simulink model "AC_FOC_PMSM_Developing_Rev_5"  (R2023b)
settings: Solver=VariableStepAuto  StartTime=0.0  StopTime=1  MaxStep=1e-4  RelTol=1e-3
values from neighbouring files (symbols this model uses):
  B = 11e-5    (= 0.00011)    [AB_FOC_For_PMSM_Parameters.m]
  Id_ref = 0    [AB_FOC_For_PMSM_Parameters.m]
  J = 0.47e-4    (= 4.7e-05)    [AB_FOC_For_PMSM_Parameters.m]
  Kcq = (2*zeta*wn*L) - Rs    (= 84.52)    [AB_FOC_For_PMSM_Parameters.m]
  Kcs = ((2*zeta*wns) - (B/J)) / ((1.5 *(pole^2)*flux)/J)    (= 0.00768666666667)    [AB_FOC_For_PMSM_Parameters.m]
  Ld = 7e-2    (= 0.07)    [AB_FOC_For_PMSM_Parameters.m]
  Lq = 7e-2    (= 0.07)    [AB_FOC_For_PMSM_Parameters.m]
  pole = 2    [AB_FOC_For_PMSM_Parameters.m]
  Rs = 2.98    [AB_FOC_For_PMSM_Parameters.m]
  speed_ref = 500    [AB_FOC_For_PMSM_Parameters.m]
libraries: fuzblock x10, slpidlib x9, spsDCVoltageSourceLib x5, spsPermanentMagnetSynchronousMachineLib x5, spsThreePhaseVIMeasurementLib x5, spsUniversalBridgeLib x5, spsdq0toabcLib x1, sps_lib x1
(part 1 of 2)
settings Model: Creator=hkurt  LastModifiedBy=hkurt
settings SolverCC: ZeroCrossAlgorithm=Adaptive

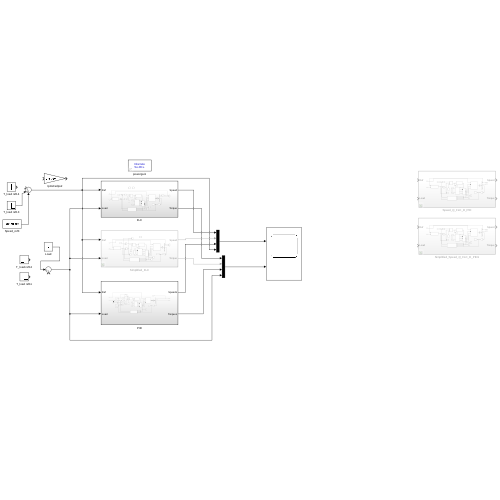
[thumbnail: Simulink's stored preview of the top-level diagram]
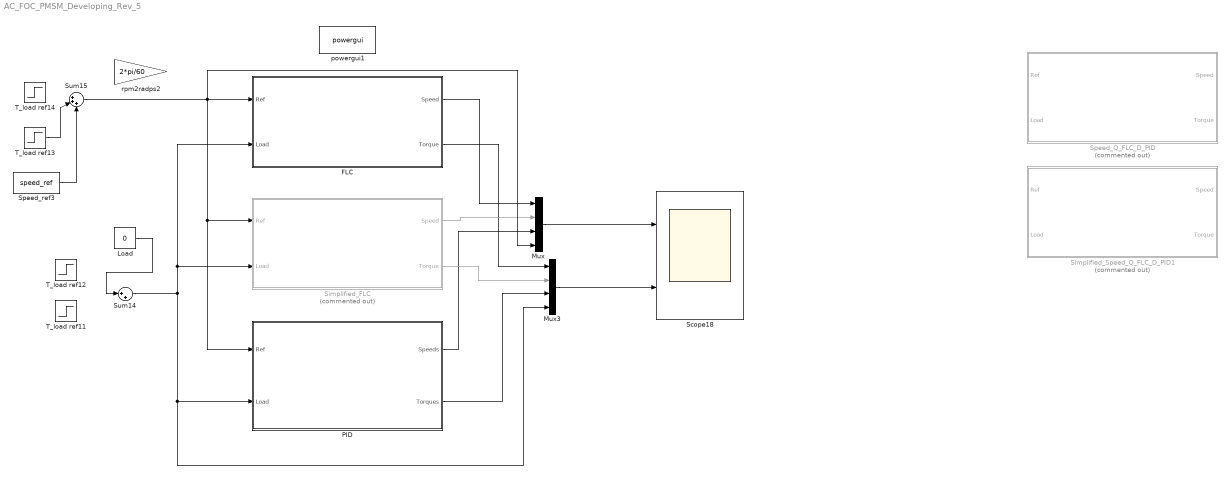
== system AC_FOC_PMSM_Developing_Rev_5 ==
  FLC : Subsystem
  Load : Constant  Value=0
  Mux : Mux
  Mux3 : Mux
  PID : Subsystem
  Scope18 : Scope  NumInputPorts=2
  Simplified_FLC : Subsystem  Commented=on
  Simplified_Speed_Q_FLC_D_PID1 : Subsystem  Commented=on
  Speed_Q_FLC_D_PID : Subsystem  Commented=on
  Speed_ref3 : Constant  Value=speed_ref
  Sum14 : Sum  Inputs=|++
  Sum15 : Sum  Inputs=|+++
  T_load ref11 : Step  Time=0.8  After=-0.1  SampleTime=0
  T_load ref12 : Step  Time=0.6  After=0.2  SampleTime=0
  T_load ref13 : Step  Time=0.5  After=-400  SampleTime=0
  T_load ref14 : Step  Time=0.2  After=300  SampleTime=0
  powergui1 : sps_lib/powergui  Priority=1  SimulationMode=Discrete  SampleTime=50e-7  frequency=60  Iterations=50  frequencyindice=0  Pbase=100e6  ErrMax=1e-4  UnitsV=kV  UnitsW=MW  buscounter=0  FunctionMessages=off  echomessages=off  EnableUseOfTLC=off  CurrentSourceSwitches=off  DisableSnubberDevices=off  DisableRonSwitches=off  DisableVfSwitches=off  DisplayEquations=off  AutomaticDiscreteSolvers=off  SolverType=Tustin/Backward Euler (TBE)  Interpol=off  ExternalGateDelay=off  methode=off  Ts=100  x0status=blocks  SPID=on  SwTol=0  HookPort=off  NonlinearTolerance=1e-4  nMaxIteration=100  ContinueOnMaxIteration=off  RestoreLinks=warning  ResistiveCurrentMeasurement=off  Frange=[0:2:500]  Ylog=off  Xlog=on  ShowGrid=off  save=off  variable=ZData  structure=0  ZoomFFT=off  StartTime=0.0  cycles=1  DisplayStyle=1  fundamental=60  FreqAxis=off  MaxFrequency=1000  frequencyindicesteady=1  RmsSteady=1  display=off
  rpm2radps2 : Gain  Gain=2*pi/60
  wires:
  Speed_ref3/1 -> Sum15/3
  Sum14/1 -> Simplified_FLC/2(Load), FLC/2(Load), Mux3/4, PID/2(Load)
  Mux/1 -> Scope18/1
  Mux3/1 -> Scope18/2
  PID/1(Speeds) -> Mux/3
  PID/2(Torques) -> Mux3/3
  FLC/1(Speed) -> Mux/1
  FLC/2(Torque) -> Mux3/1
  Simplified_FLC/1(Speed) -> Mux/2
  Simplified_FLC/2(Torque) -> Mux3/2
  Load/1 -> Sum14/1
  Sum15/1 -> Mux/4, PID/1(Ref), Simplified_FLC/1(Ref), FLC/1(Ref)
  T_load ref13/1 -> Sum15/2

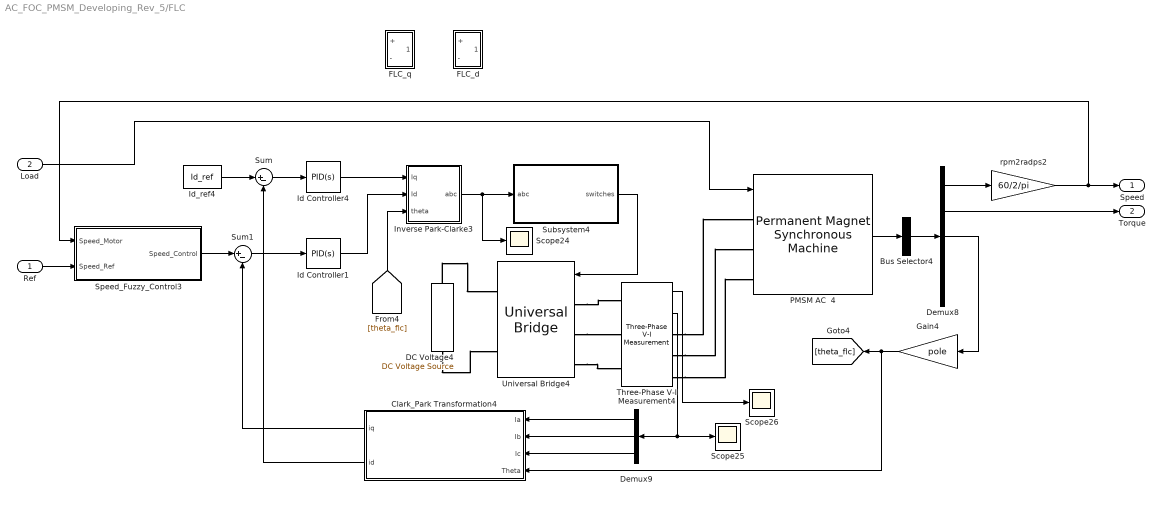
== system AC_FOC_PMSM_Developing_Rev_5/FLC ==
  Ref : Inport
  Load : Inport  Port=2
  Bus Selector4 : BusSelector  OutputSignals=Rotor speed wm (rad/s),Electromagnetic torque Te (N*m),Rotor angle thetam (rad),Stator current is_q (A),Stator current is_d (A)  OutputAsBus=on
  Clark_Park Transformation4 : Subsystem
  DC Voltage4 : spsDCVoltageSourceLib/DC Voltage Source  Amplitude=600  Measurements=None
  Demux8 : Demux  Outputs=5
  Demux9 : Demux  Outputs=3
  FLC_d : Subsystem
  FLC_q : Subsystem
  Gain4 : Gain  Gain=pole
  Id Controller1 : slpidlib/PID Controller  Controller=PID  Form=Parallel  TimeDomain=Continuous-time  UseExternalTs=off  SampleTime=-1  IntegratorMethod=Forward Euler  FilterMethod=Forward Euler  ControllerParametersSource=internal  P=Kcq  I=Kcq/0.001  UseKiTs=off  D=0  N=100  UseFilter=on  TunerSelectOption=Transfer Function Based (PID Tuner App)  InitialConditionSource=internal  InitialConditionForIntegrator=0  InitialConditionForFilter=0  DifferentiatorICPrevScaledInput=0  ExternalReset=none  TrackingMode=off  Kt=1  LimitOutput=off  SatLimitsSource=internal  UpperSaturationLimit=inf  LowerSaturationLimit=-inf  LinearizeAsGain=on  AntiWindupMode=none  Kb=1  LimitIntegrator=off  UpperIntegratorSaturationLimit=inf  LowerIntegratorSaturationLimit=-inf  POutMin=[]  POutMax=[]  IOutMin=[]  IOutMax=[]  DOutMin=[]  DOutMax=[]  NOutMin=[]  NOutMax=[]  SumOutMin=[]  SumOutMax=[]  SaturationOutMin=[]  SaturationOutMax=[]  PParamMin=[]  PParamMax=[]  IParamMin=[]  IParamMax=[]  DParamMin=[]  DParamMax=[]  NParamMin=[]  NParamMax=[]  KbParamMin=[]  KbParamMax=[]  KtParamMin=[]  KtParamMax=[]  KbOutMin=[]  KbOutMax=[]  KtOutMin=[]  KtOutMax=[]  IntegratorOutMin=[]  IntegratorOutMax=[]  FilterOutMin=[]  FilterOutMax=[]  SumI1OutMin=[]  SumI1OutMax=[]  SumI2OutMin=[]  SumI2OutMax=[]  SumI3OutMin=[]  SumI3OutMax=[]  SumI4OutMin=[]  SumI4OutMax=[]  SumDOutMin=[]  SumDOutMax=[]  DifferentiatorOutMin=[]  DifferentiatorOutMax=[]  FilterDiffOutCoefMin=[]  FilterDiffOutCoefMax=[]  ReciprocalOutMin=[]  ReciprocalOutMax=[]  SumDenOutMin=[]  SumDenOutMax=[]  SumNumOutMin=[]  SumNumOutMax=[]  DivideOutMin=[]  DivideOutMax=[]  UdiffTsProdOutMin=[]  UdiffTsProdOutMax=[]  NTsProdOutMin=[]  NTsProdOutMax=[]  UintegralTsProdOutMin=[]  UintegralTsProdOutMax=[]  UngainTsProdOutMin=[]  UngainTsProdOutMax=[]  ClampingZeroOutDataTypeStr=Inherit: Inherit via back propagation  ClampingZeroOutMin=[]  ClampingZeroOutMax=[]  FilterDenConstantOutDataTypeStr=Inherit: Inherit via back propagation  FilterDenConstantOutMin=[]  FilterDenConstantOutMax=[]  PCopyOutDataTypeStr=Inherit: Inherit via back propagation  PCopyOutMin=[]  PCopyOutMax=[]  NCopyOutDataTypeStr=Inherit: Inherit via back propagation  NCopyOutMin=[]  NCopyOutMax=[]  IntegratorContinuousStateAttributes=''  IntegratorStateMustResolveToSignalObject=off  IntegratorRTWStateStorageClass=Auto  FilterContinuousStateAttributes=''  FilterStateMustResolveToSignalObject=off  FilterRTWStateStorageClass=Auto  ParallelPVariant=InternalParameters  IdealPVariant=Disabled  IVariant=InternalParameters  DVariant=InternalParameters  IntegratorVariant=Continuous  SatVariant=Disabled  AWVariant=Passthrough  PCopyVariant=Disabled  TRVariant=Disabled  FdbkBlocksVariant=Forward  IdealPFdbkVariant=Disabled  SatFdbkVariant=Disabled  DerivativeFilterVariant=ContFilter  NVariant=InternalParameters  NCopyVariant=Disabled  FilterICVariant=InternalICsFilter  IntegratorICVariant=InternalICs  ExternalResetVariant=Disabled  TRSumVariant=Passthrough  SumFdbkVariant=Disabled  SumVariant=Sum_PID  TsampFilterVariant=InternalTs  TsampNgainVariant=Passthrough  TsampIntegralVariant=Disabled_SignalSpec  ExternalSaturationOutDataTypeStr=Inherit: Same as second input
  Id Controller4 : slpidlib/PID Controller  Controller=PID  Form=Parallel  TimeDomain=Continuous-time  UseExternalTs=off  SampleTime=-1  IntegratorMethod=Forward Euler  FilterMethod=Forward Euler  ControllerParametersSource=internal  P=Kcq  I=Kcq/0.001  UseKiTs=off  D=0  N=100  UseFilter=on  TunerSelectOption=Transfer Function Based (PID Tuner App)  InitialConditionSource=internal  InitialConditionForIntegrator=0  InitialConditionForFilter=0  DifferentiatorICPrevScaledInput=0  ExternalReset=none  TrackingMode=off  Kt=1  LimitOutput=off  SatLimitsSource=internal  UpperSaturationLimit=inf  LowerSaturationLimit=-inf  LinearizeAsGain=on  AntiWindupMode=none  Kb=1  LimitIntegrator=off  UpperIntegratorSaturationLimit=inf  LowerIntegratorSaturationLimit=-inf  POutMin=[]  POutMax=[]  IOutMin=[]  IOutMax=[]  DOutMin=[]  DOutMax=[]  NOutMin=[]  NOutMax=[]  SumOutMin=[]  SumOutMax=[]  SaturationOutMin=[]  SaturationOutMax=[]  PParamMin=[]  PParamMax=[]  IParamMin=[]  IParamMax=[]  DParamMin=[]  DParamMax=[]  NParamMin=[]  NParamMax=[]  KbParamMin=[]  KbParamMax=[]  KtParamMin=[]  KtParamMax=[]  KbOutMin=[]  KbOutMax=[]  KtOutMin=[]  KtOutMax=[]  IntegratorOutMin=[]  IntegratorOutMax=[]  FilterOutMin=[]  FilterOutMax=[]  SumI1OutMin=[]  SumI1OutMax=[]  SumI2OutMin=[]  SumI2OutMax=[]  SumI3OutMin=[]  SumI3OutMax=[]  SumI4OutMin=[]  SumI4OutMax=[]  SumDOutMin=[]  SumDOutMax=[]  DifferentiatorOutMin=[]  DifferentiatorOutMax=[]  FilterDiffOutCoefMin=[]  FilterDiffOutCoefMax=[]  ReciprocalOutMin=[]  ReciprocalOutMax=[]  SumDenOutMin=[]  SumDenOutMax=[]  SumNumOutMin=[]  SumNumOutMax=[]  DivideOutMin=[]  DivideOutMax=[]  UdiffTsProdOutMin=[]  UdiffTsProdOutMax=[]  NTsProdOutMin=[]  NTsProdOutMax=[]  UintegralTsProdOutMin=[]  UintegralTsProdOutMax=[]  UngainTsProdOutMin=[]  UngainTsProdOutMax=[]  ClampingZeroOutDataTypeStr=Inherit: Inherit via back propagation  ClampingZeroOutMin=[]  ClampingZeroOutMax=[]  FilterDenConstantOutDataTypeStr=Inherit: Inherit via back propagation  FilterDenConstantOutMin=[]  FilterDenConstantOutMax=[]  PCopyOutDataTypeStr=Inherit: Inherit via back propagation  PCopyOutMin=[]  PCopyOutMax=[]  NCopyOutDataTypeStr=Inherit: Inherit via back propagation  NCopyOutMin=[]  NCopyOutMax=[]  IntegratorContinuousStateAttributes=''  IntegratorStateMustResolveToSignalObject=off  IntegratorRTWStateStorageClass=Auto  FilterContinuousStateAttributes=''  FilterStateMustResolveToSignalObject=off  FilterRTWStateStorageClass=Auto  ParallelPVariant=InternalParameters  IdealPVariant=Disabled  IVariant=InternalParameters  DVariant=InternalParameters  IntegratorVariant=Continuous  SatVariant=Disabled  AWVariant=Passthrough  PCopyVariant=Disabled  TRVariant=Disabled  FdbkBlocksVariant=Forward  IdealPFdbkVariant=Disabled  SatFdbkVariant=Disabled  DerivativeFilterVariant=ContFilter  NVariant=InternalParameters  NCopyVariant=Disabled  FilterICVariant=InternalICsFilter  IntegratorICVariant=InternalICs  ExternalResetVariant=Disabled  TRSumVariant=Passthrough  SumFdbkVariant=Disabled  SumVariant=Sum_PID  TsampFilterVariant=InternalTs  TsampNgainVariant=Passthrough  TsampIntegralVariant=Disabled_SignalSpec  ExternalSaturationOutDataTypeStr=Inherit: Same as second input
  Id_ref4 : Constant  Value=Id_ref
  Inverse Park-Clarke3 : Subsystem
  PMSM AC  4 : spsPermanentMagnetSynchronousMachineLib/Permanent Magnet Synchronous Machine  NbPhases=3  FluxDistribution=Sinusoidal  RotorType=Round  MechanicalLoad=Torque Tm  PresetModel=No  ShowDetailedParameters=on  MeasurementBus=off  Resistance=Rs  Inductance=8.5e-3  dqInductances=[Ld, Lq]  La=0.000395  MachineConstant=Flux linkage established by magnets (V.s)  Flux=flux  VoltageCst=45.345  TorqueCst=0.375  Flat=120  Mechanical=[J B pole 0]  PolePairs=4  InitialConditions=[0,0, 0,0]  InitialConditions5ph=[0 0 0 0 0 0]  RefAngle=90 degrees behind phase A axis (modified Park)  IterativeDiscreteModel=Trapezoidal non iterative  TsBlock=-1  TsPowergui=0
  Scope24 : Scope
  Scope25 : Scope
  Scope26 : Scope
  Speed_Fuzzy_Control3 : Subsystem
  Subsystem4 : Subsystem
  Sum : Sum  Inputs=|+-
  Sum1 : Sum  Inputs=|+-
  Three-Phase V-I Measurement4 : spsThreePhaseVIMeasurementLib/Three-Phase V-I Measurement  VoltageMeasurement=phase-to-phase  SetLabelV=off  LabelV=Vabc  Vpu=off  VpuLL=off  CurrentMeasurement=yes  SetLabelI=off  LabelI=Iabc  Ipu=off  Pbase=100e6  Vbase=500e3  OutputType=Complex  PhasorSimulation=off  PSBequivalent=0
  Universal Bridge4 : spsUniversalBridgeLib/Universal Bridge  Arms=3  SnubberResistance=1e5  SnubberCapacitance=inf  Device=IGBT / Diodes  Ron=1e-3  Lon=0  ForwardVoltages="[  0  0  ]"  ForwardVoltage=0  GTOparameters=[ 10e-6 , 20e-6 ]  IGBTparameters=[ 1e-6 , 2e-6 ]  Measurements=None  Measurements_2=None  converterType=Rectifier
  rpm2radps2 : Gain  Gain=60/2/pi
  Speed : Outport
  Torque : Outport  Port=2
  wires:
  Three-Phase V-I Measurement4/2 -> Demux9/1, Scope25/1
  Subsystem4/1(switches) -> Universal Bridge4/1
  Three-Phase V-I Measurement4/1 -> Scope26/1
  Demux8/2 -> Torque/1
  Inverse Park-Clarke3/1(abc) -> Scope24/1, Subsystem4/1(abc)
  Bus Selector4/1 -> Demux8/1
  Demux9/2 -> Clark_Park Transformation4/2(Ib)
  [theta_flc] -> Inverse Park-Clarke3/3(theta)
  Ref/1 -> Speed_Fuzzy_Control3/2(Speed_Ref)
  Gain4/1 -> Clark_Park Transformation4/4(Theta), [theta_flc]
  Demux9/1 -> Clark_Park Transformation4/1(Ia)
  Demux9/3 -> Clark_Park Transformation4/3(Ic)
  Demux8/3 -> Gain4/1
  PMSM AC  4/1 -> Bus Selector4/1
  Load/1 -> PMSM AC  4/1
  Demux8/1 -> rpm2radps2/1
  Id Controller4/1 -> Inverse Park-Clarke3/1(Iq)
  Sum/1 -> Id Controller4/1
  Clark_Park Transformation4/2(id) -> Sum/2
  Id_ref4/1 -> Sum/1
  Speed_Fuzzy_Control3/1(Speed_Control) -> Sum1/1
  Sum1/1 -> Id Controller1/1
  Id Controller1/1 -> Inverse Park-Clarke3/2(Id)
  Clark_Park Transformation4/1(iq) -> Sum1/2
  rpm2radps2/1 -> Speed/1, Speed_Fuzzy_Control3/1(Speed_Motor)
  connections:
  DC Voltage4/LConn1 -- Universal Bridge4/RConn2
  Universal Bridge4/LConn2 -- Three-Phase V-I Measurement4/LConn2
  Three-Phase V-I Measurement4/RConn2 -- PMSM AC  4/LConn2
  Universal Bridge4/LConn3 -- Three-Phase V-I Measurement4/LConn3
  DC Voltage4/RConn1 -- Universal Bridge4/RConn1
  Universal Bridge4/LConn1 -- Three-Phase V-I Measurement4/LConn1
  Three-Phase V-I Measurement4/RConn3 -- PMSM AC  4/LConn3
  Three-Phase V-I Measurement4/RConn1 -- PMSM AC  4/LConn1

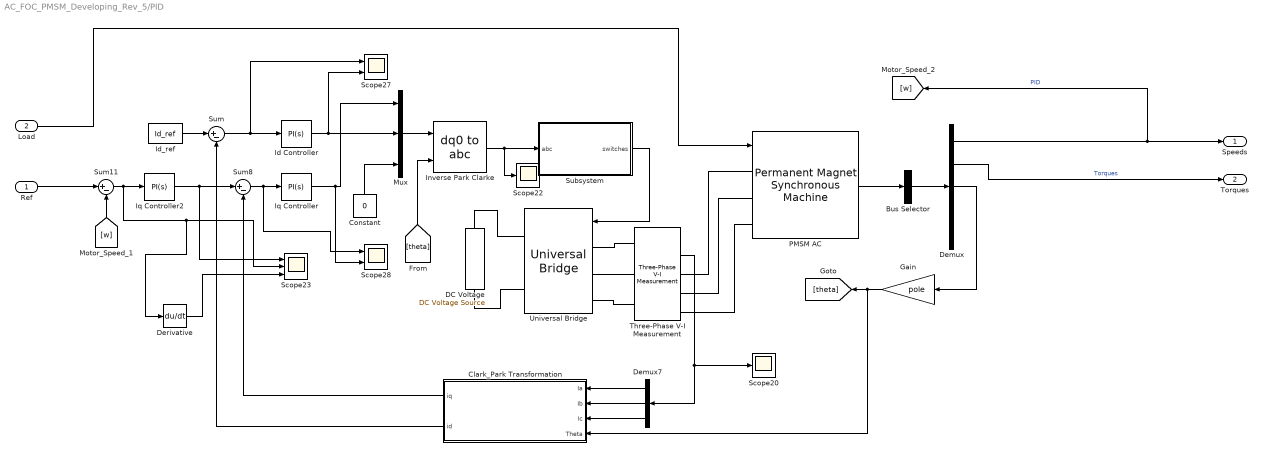
== system AC_FOC_PMSM_Developing_Rev_5/PID ==
  Ref : Inport
  Load : Inport  Port=2
  Bus Selector : BusSelector  OutputSignals=Rotor speed wm (rad/s),Electromagnetic torque Te (N*m),Rotor angle thetam (rad),Stator current is_q (A),Stator current is_d (A)  OutputAsBus=on
  Clark_Park Transformation : Subsystem
  Constant : Constant  Value=0
  DC Voltage : spsDCVoltageSourceLib/DC Voltage Source  Amplitude=600  Measurements=None
  Demux : Demux  Outputs=5
  Demux7 : Demux  Outputs=3
  Derivative : Derivative
  Gain : Gain  Gain=pole
  Id Controller : slpidlib/PID Controller  Controller=PI  Form=Parallel  TimeDomain=Continuous-time  UseExternalTs=off  SampleTime=-1  IntegratorMethod=Forward Euler  FilterMethod=Forward Euler  ControllerParametersSource=internal  P=Kcq  I=Kcq/0.001  UseKiTs=off  D=0  N=100  UseFilter=on  TunerSelectOption=Transfer Function Based (PID Tuner App)  InitialConditionSource=internal  InitialConditionForIntegrator=0  InitialConditionForFilter=0  DifferentiatorICPrevScaledInput=0  ExternalReset=none  TrackingMode=off  Kt=1  LimitOutput=off  SatLimitsSource=internal  UpperSaturationLimit=inf  LowerSaturationLimit=-inf  LinearizeAsGain=on  AntiWindupMode=none  Kb=1  LimitIntegrator=off  UpperIntegratorSaturationLimit=inf  LowerIntegratorSaturationLimit=-inf  POutMin=[]  POutMax=[]  IOutMin=[]  IOutMax=[]  DOutMin=[]  DOutMax=[]  NOutMin=[]  NOutMax=[]  SumOutMin=[]  SumOutMax=[]  SaturationOutMin=[]  SaturationOutMax=[]  PParamMin=[]  PParamMax=[]  IParamMin=[]  IParamMax=[]  DParamMin=[]  DParamMax=[]  NParamMin=[]  NParamMax=[]  KbParamMin=[]  KbParamMax=[]  KtParamMin=[]  KtParamMax=[]  KbOutMin=[]  KbOutMax=[]  KtOutMin=[]  KtOutMax=[]  IntegratorOutMin=[]  IntegratorOutMax=[]  FilterOutMin=[]  FilterOutMax=[]  SumI1OutMin=[]  SumI1OutMax=[]  SumI2OutMin=[]  SumI2OutMax=[]  SumI3OutMin=[]  SumI3OutMax=[]  SumI4OutMin=[]  SumI4OutMax=[]  SumDOutMin=[]  SumDOutMax=[]  DifferentiatorOutMin=[]  DifferentiatorOutMax=[]  FilterDiffOutCoefMin=[]  FilterDiffOutCoefMax=[]  ReciprocalOutMin=[]  ReciprocalOutMax=[]  SumDenOutMin=[]  SumDenOutMax=[]  SumNumOutMin=[]  SumNumOutMax=[]  DivideOutMin=[]  DivideOutMax=[]  UdiffTsProdOutMin=[]  UdiffTsProdOutMax=[]  NTsProdOutMin=[]  NTsProdOutMax=[]  UintegralTsProdOutMin=[]  UintegralTsProdOutMax=[]  UngainTsProdOutMin=[]  UngainTsProdOutMax=[]  ClampingZeroOutDataTypeStr=Inherit: Inherit via back propagation  ClampingZeroOutMin=[]  ClampingZeroOutMax=[]  FilterDenConstantOutDataTypeStr=Inherit: Inherit via back propagation  FilterDenConstantOutMin=[]  FilterDenConstantOutMax=[]  PCopyOutDataTypeStr=Inherit: Inherit via back propagation  PCopyOutMin=[]  PCopyOutMax=[]  NCopyOutDataTypeStr=Inherit: Inherit via back propagation  NCopyOutMin=[]  NCopyOutMax=[]  IntegratorContinuousStateAttributes=''  IntegratorStateMustResolveToSignalObject=off  IntegratorRTWStateStorageClass=Auto  FilterContinuousStateAttributes=''  FilterStateMustResolveToSignalObject=off  FilterRTWStateStorageClass=Auto  ParallelPVariant=InternalParameters  IdealPVariant=Disabled  IVariant=InternalParameters  DVariant=Disabled  IntegratorVariant=Continuous  SatVariant=Disabled  AWVariant=Passthrough  PCopyVariant=Disabled  TRVariant=Disabled  FdbkBlocksVariant=Forward  IdealPFdbkVariant=Disabled  SatFdbkVariant=Disabled  DerivativeFilterVariant=Disabled  NVariant=Disabled  NCopyVariant=Disabled_SignalSpec  FilterICVariant=Disabled  IntegratorICVariant=InternalICs  ExternalResetVariant=Disabled  TRSumVariant=Passthrough  SumFdbkVariant=Disabled  SumVariant=Sum_PI  TsampFilterVariant=InternalTs  TsampNgainVariant=Passthrough  TsampIntegralVariant=Disabled_SignalSpec  ExternalSaturationOutDataTypeStr=Inherit: Same as second input
  Id_ref : Constant  Value=Id_ref
  Inverse Park Clarke : spsdq0toabcLib/dq0 to abc  Alignment=Aligned with phase A axis
  Iq Controller : slpidlib/PID Controller  Controller=PI  Form=Parallel  TimeDomain=Continuous-time  UseExternalTs=off  SampleTime=-1  IntegratorMethod=Forward Euler  FilterMethod=Forward Euler  ControllerParametersSource=internal  P=Kcq  I=Kcq/0.001  UseKiTs=off  D=0  N=100  UseFilter=on  TunerSelectOption=Transfer Function Based (PID Tuner App)  InitialConditionSource=internal  InitialConditionForIntegrator=0  InitialConditionForFilter=0  DifferentiatorICPrevScaledInput=0  ExternalReset=none  TrackingMode=off  Kt=1  LimitOutput=off  SatLimitsSource=internal  UpperSaturationLimit=inf  LowerSaturationLimit=-inf  LinearizeAsGain=on  AntiWindupMode=none  Kb=1  LimitIntegrator=off  UpperIntegratorSaturationLimit=inf  LowerIntegratorSaturationLimit=-inf  POutMin=[]  POutMax=[]  IOutMin=[]  IOutMax=[]  DOutMin=[]  DOutMax=[]  NOutMin=[]  NOutMax=[]  SumOutMin=[]  SumOutMax=[]  SaturationOutMin=[]  SaturationOutMax=[]  PParamMin=[]  PParamMax=[]  IParamMin=[]  IParamMax=[]  DParamMin=[]  DParamMax=[]  NParamMin=[]  NParamMax=[]  KbParamMin=[]  KbParamMax=[]  KtParamMin=[]  KtParamMax=[]  KbOutMin=[]  KbOutMax=[]  KtOutMin=[]  KtOutMax=[]  IntegratorOutMin=[]  IntegratorOutMax=[]  FilterOutMin=[]  FilterOutMax=[]  SumI1OutMin=[]  SumI1OutMax=[]  SumI2OutMin=[]  SumI2OutMax=[]  SumI3OutMin=[]  SumI3OutMax=[]  SumI4OutMin=[]  SumI4OutMax=[]  SumDOutMin=[]  SumDOutMax=[]  DifferentiatorOutMin=[]  DifferentiatorOutMax=[]  FilterDiffOutCoefMin=[]  FilterDiffOutCoefMax=[]  ReciprocalOutMin=[]  ReciprocalOutMax=[]  SumDenOutMin=[]  SumDenOutMax=[]  SumNumOutMin=[]  SumNumOutMax=[]  DivideOutMin=[]  DivideOutMax=[]  UdiffTsProdOutMin=[]  UdiffTsProdOutMax=[]  NTsProdOutMin=[]  NTsProdOutMax=[]  UintegralTsProdOutMin=[]  UintegralTsProdOutMax=[]  UngainTsProdOutMin=[]  UngainTsProdOutMax=[]  ClampingZeroOutDataTypeStr=Inherit: Inherit via back propagation  ClampingZeroOutMin=[]  ClampingZeroOutMax=[]  FilterDenConstantOutDataTypeStr=Inherit: Inherit via back propagation  FilterDenConstantOutMin=[]  FilterDenConstantOutMax=[]  PCopyOutDataTypeStr=Inherit: Inherit via back propagation  PCopyOutMin=[]  PCopyOutMax=[]  NCopyOutDataTypeStr=Inherit: Inherit via back propagation  NCopyOutMin=[]  NCopyOutMax=[]  IntegratorContinuousStateAttributes=''  IntegratorStateMustResolveToSignalObject=off  IntegratorRTWStateStorageClass=Auto  FilterContinuousStateAttributes=''  FilterStateMustResolveToSignalObject=off  FilterRTWStateStorageClass=Auto  ParallelPVariant=InternalParameters  IdealPVariant=Disabled  IVariant=InternalParameters  DVariant=Disabled  IntegratorVariant=Continuous  SatVariant=Disabled  AWVariant=Passthrough  PCopyVariant=Disabled  TRVariant=Disabled  FdbkBlocksVariant=Forward  IdealPFdbkVariant=Disabled  SatFdbkVariant=Disabled  DerivativeFilterVariant=Disabled  NVariant=Disabled  NCopyVariant=Disabled_SignalSpec  FilterICVariant=Disabled  IntegratorICVariant=InternalICs  ExternalResetVariant=Disabled  TRSumVariant=Passthrough  SumFdbkVariant=Disabled  SumVariant=Sum_PI  TsampFilterVariant=InternalTs  TsampNgainVariant=Passthrough  TsampIntegralVariant=Disabled_SignalSpec  ExternalSaturationOutDataTypeStr=Inherit: Same as second input
  Iq Controller2 : slpidlib/PID Controller  Controller=PI  Form=Parallel  TimeDomain=Continuous-time  UseExternalTs=off  SampleTime=-1  IntegratorMethod=Forward Euler  FilterMethod=Forward Euler  ControllerParametersSource=internal  P=Kcs  I=Kcs/0.2001  UseKiTs=off  D=0  N=100  UseFilter=on  TunerSelectOption=Transfer Function Based (PID Tuner App)  InitialConditionSource=internal  InitialConditionForIntegrator=0  InitialConditionForFilter=0  DifferentiatorICPrevScaledInput=0  ExternalReset=none  TrackingMode=off  Kt=1  LimitOutput=off  SatLimitsSource=internal  UpperSaturationLimit=inf  LowerSaturationLimit=-inf  LinearizeAsGain=on  AntiWindupMode=none  Kb=1  LimitIntegrator=off  UpperIntegratorSaturationLimit=inf  LowerIntegratorSaturationLimit=-inf  POutMin=[]  POutMax=[]  IOutMin=[]  IOutMax=[]  DOutMin=[]  DOutMax=[]  NOutMin=[]  NOutMax=[]  SumOutMin=[]  SumOutMax=[]  SaturationOutMin=[]  SaturationOutMax=[]  PParamMin=[]  PParamMax=[]  IParamMin=[]  IParamMax=[]  DParamMin=[]  DParamMax=[]  NParamMin=[]  NParamMax=[]  KbParamMin=[]  KbParamMax=[]  KtParamMin=[]  KtParamMax=[]  KbOutMin=[]  KbOutMax=[]  KtOutMin=[]  KtOutMax=[]  IntegratorOutMin=[]  IntegratorOutMax=[]  FilterOutMin=[]  FilterOutMax=[]  SumI1OutMin=[]  SumI1OutMax=[]  SumI2OutMin=[]  SumI2OutMax=[]  SumI3OutMin=[]  SumI3OutMax=[]  SumI4OutMin=[]  SumI4OutMax=[]  SumDOutMin=[]  SumDOutMax=[]  DifferentiatorOutMin=[]  DifferentiatorOutMax=[]  FilterDiffOutCoefMin=[]  FilterDiffOutCoefMax=[]  ReciprocalOutMin=[]  ReciprocalOutMax=[]  SumDenOutMin=[]  SumDenOutMax=[]  SumNumOutMin=[]  SumNumOutMax=[]  DivideOutMin=[]  DivideOutMax=[]  UdiffTsProdOutMin=[]  UdiffTsProdOutMax=[]  NTsProdOutMin=[]  NTsProdOutMax=[]  UintegralTsProdOutMin=[]  UintegralTsProdOutMax=[]  UngainTsProdOutMin=[]  UngainTsProdOutMax=[]  ClampingZeroOutDataTypeStr=Inherit: Inherit via back propagation  ClampingZeroOutMin=[]  ClampingZeroOutMax=[]  FilterDenConstantOutDataTypeStr=Inherit: Inherit via back propagation  FilterDenConstantOutMin=[]  FilterDenConstantOutMax=[]  PCopyOutDataTypeStr=Inherit: Inherit via back propagation  PCopyOutMin=[]  PCopyOutMax=[]  NCopyOutDataTypeStr=Inherit: Inherit via back propagation  NCopyOutMin=[]  NCopyOutMax=[]  IntegratorContinuousStateAttributes=''  IntegratorStateMustResolveToSignalObject=off  IntegratorRTWStateStorageClass=Auto  FilterContinuousStateAttributes=''  FilterStateMustResolveToSignalObject=off  FilterRTWStateStorageClass=Auto  ParallelPVariant=InternalParameters  IdealPVariant=Disabled  IVariant=InternalParameters  DVariant=Disabled  IntegratorVariant=Continuous  SatVariant=Disabled  AWVariant=Passthrough  PCopyVariant=Disabled  TRVariant=Disabled  FdbkBlocksVariant=Forward  IdealPFdbkVariant=Disabled  SatFdbkVariant=Disabled  DerivativeFilterVariant=Disabled  NVariant=Disabled  NCopyVariant=Disabled_SignalSpec  FilterICVariant=Disabled  IntegratorICVariant=InternalICs  ExternalResetVariant=Disabled  TRSumVariant=Passthrough  SumFdbkVariant=Disabled  SumVariant=Sum_PI  TsampFilterVariant=InternalTs  TsampNgainVariant=Passthrough  TsampIntegralVariant=Disabled_SignalSpec  ExternalSaturationOutDataTypeStr=Inherit: Same as second input
  Mux : Mux  Inputs=3
  "PMSM AC  " : spsPermanentMagnetSynchronousMachineLib/Permanent Magnet Synchronous Machine  NbPhases=3  FluxDistribution=Sinusoidal  RotorType=Salient-pole  MechanicalLoad=Torque Tm  PresetModel=No  ShowDetailedParameters=on  MeasurementBus=off  Resistance=Rs  Inductance=8.5e-3  dqInductances=[Ld, Lq]  La=0.000395  MachineConstant=Flux linkage established by magnets (V.s)  Flux=flux  VoltageCst=280.7761  TorqueCst=2.322  Flat=120  Mechanical=[J B pole 0]  PolePairs=4  InitialConditions=[0,0, 0,0]  InitialConditions5ph=[0 0 0 0 0 0]  RefAngle=90 degrees behind phase A axis (modified Park)  IterativeDiscreteModel=Trapezoidal non iterative  TsBlock=-1  TsPowergui=0
  Scope20 : Scope
  Scope22 : Scope
  Scope23 : Scope  NumInputPorts=3
  Scope27 : Scope  NumInputPorts=2
  Scope28 : Scope  NumInputPorts=2
  Subsystem : Subsystem
  Sum : Sum  Inputs=|+-
  Sum11 : Sum  Inputs=|+-
  Sum8 : Sum  Inputs=|+-
  Three-Phase V-I Measurement : spsThreePhaseVIMeasurementLib/Three-Phase V-I Measurement  VoltageMeasurement=phase-to-phase  SetLabelV=off  LabelV=Vabc  Vpu=off  VpuLL=off  CurrentMeasurement=yes  SetLabelI=off  LabelI=Iabc  Ipu=off  Pbase=100e6  Vbase=500e3  OutputType=Complex  PhasorSimulation=off  PSBequivalent=0
  Universal Bridge : spsUniversalBridgeLib/Universal Bridge  Arms=3  SnubberResistance=1e5  SnubberCapacitance=inf  Device=IGBT / Diodes  Ron=1e-3  Lon=0  ForwardVoltages="[  0  0  ]"  ForwardVoltage=0  GTOparameters=[ 10e-6 , 20e-6 ]  IGBTparameters=[ 1e-6 , 2e-6 ]  Measurements=None  Measurements_2=None  converterType=Rectifier
  Speeds : Outport
  Torques : Outport  Port=2
  wires:
  Demux/3 -> Gain/1
  [theta] -> Inverse Park Clarke/2
  Sum11/1 -> Derivative/1, Scope23/2, Iq Controller2/1
  Sum8/1 -> Scope28/1, Iq Controller/1
  Demux7/3 -> Clark_Park Transformation/3(Ic)
  Iq Controller2/1 -> Scope23/1, Sum8/1
  Three-Phase V-I Measurement/2 -> Demux7/1, Scope20/1
  Gain/1 -> Clark_Park Transformation/4(Theta), [theta]
  [w] -> Sum11/2
  Clark_Park Transformation/1(iq) -> Sum8/2
  Demux7/1 -> Clark_Park Transformation/1(Ia)
  Demux/2 -> Torques/1  "Torques"
  Clark_Park Transformation/2(id) -> Sum/2
  Subsystem/1(switches) -> Universal Bridge/1
  Id Controller/1 -> Scope27/2, Mux/2
  Constant/1 -> Mux/3
  Sum/1 -> Scope27/1, Id Controller/1
  Id_ref/1 -> Sum/1
  Ref/1 -> Sum11/1
  Bus Selector/1 -> Demux/1
  Inverse Park Clarke/1 -> Scope22/1, Subsystem/1(abc)
  Mux/1 -> Inverse Park Clarke/1
  Demux/1 -> [w], Speeds/1  "PID"
  "PMSM AC  "/1 -> Bus Selector/1
  Iq Controller/1 -> Scope28/2, Mux/1
  Demux7/2 -> Clark_Park Transformation/2(Ib)
  Derivative/1 -> Scope23/3
  Load/1 -> "PMSM AC  "/1
  connections:
  Universal Bridge/LConn3 -- Three-Phase V-I Measurement/LConn3
  Three-Phase V-I Measurement/RConn2 -- "PMSM AC  "/LConn2
  Three-Phase V-I Measurement/RConn3 -- "PMSM AC  "/LConn3
  DC Voltage/LConn1 -- Universal Bridge/RConn2
  Three-Phase V-I Measurement/RConn1 -- "PMSM AC  "/LConn1
  Universal Bridge/LConn2 -- Three-Phase V-I Measurement/LConn2
  Universal Bridge/LConn1 -- Three-Phase V-I Measurement/LConn1
  DC Voltage/RConn1 -- Universal Bridge/RConn1

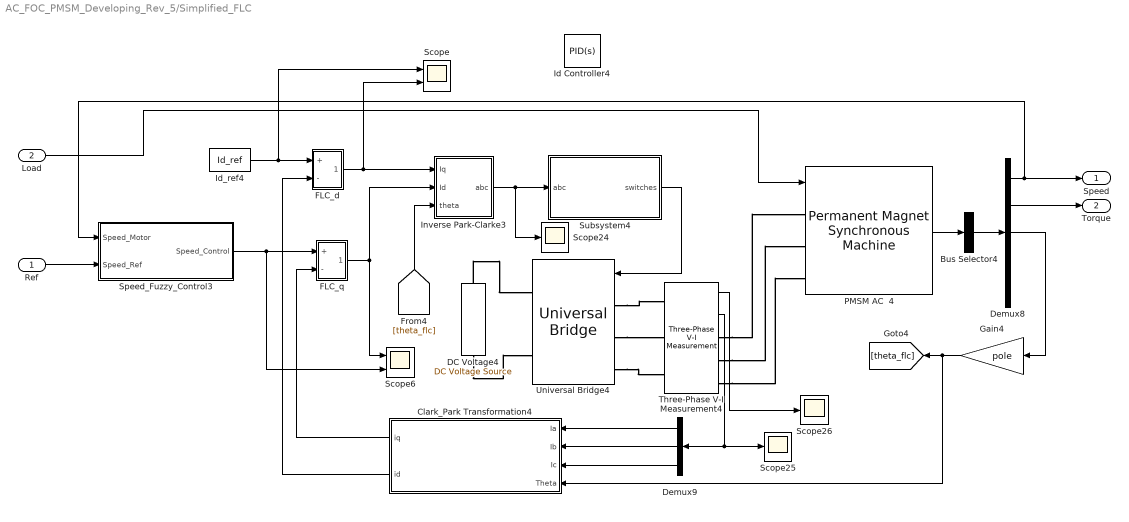
== system AC_FOC_PMSM_Developing_Rev_5/Simplified_FLC ==
  Ref : Inport
  Load : Inport  Port=2
  Bus Selector4 : BusSelector  OutputSignals=Rotor speed wm (rad/s),Electromagnetic torque Te (N*m),Rotor angle thetam (rad),Stator current is_q (A),Stator current is_d (A)  OutputAsBus=on
  Clark_Park Transformation4 : Subsystem
  DC Voltage4 : spsDCVoltageSourceLib/DC Voltage Source  Amplitude=600  Measurements=None
  Demux8 : Demux  Outputs=5
  Demux9 : Demux  Outputs=3
  FLC_d : Subsystem
  FLC_q : Subsystem
  Gain4 : Gain  Gain=pole
  Id Controller4 : slpidlib/PID Controller  Controller=PID  Form=Parallel  TimeDomain=Continuous-time  UseExternalTs=off  SampleTime=-1  IntegratorMethod=Forward Euler  FilterMethod=Forward Euler  ControllerParametersSource=internal  P=Kcq  I=Kcq/0.001  UseKiTs=off  D=0  N=100  UseFilter=on  TunerSelectOption=Transfer Function Based (PID Tuner App)  InitialConditionSource=internal  InitialConditionForIntegrator=0  InitialConditionForFilter=0  DifferentiatorICPrevScaledInput=0  ExternalReset=none  TrackingMode=off  Kt=1  LimitOutput=off  SatLimitsSource=internal  UpperSaturationLimit=inf  LowerSaturationLimit=-inf  LinearizeAsGain=on  AntiWindupMode=none  Kb=1  LimitIntegrator=off  UpperIntegratorSaturationLimit=inf  LowerIntegratorSaturationLimit=-inf  POutMin=[]  POutMax=[]  IOutMin=[]  IOutMax=[]  DOutMin=[]  DOutMax=[]  NOutMin=[]  NOutMax=[]  SumOutMin=[]  SumOutMax=[]  SaturationOutMin=[]  SaturationOutMax=[]  PParamMin=[]  PParamMax=[]  IParamMin=[]  IParamMax=[]  DParamMin=[]  DParamMax=[]  NParamMin=[]  NParamMax=[]  KbParamMin=[]  KbParamMax=[]  KtParamMin=[]  KtParamMax=[]  KbOutMin=[]  KbOutMax=[]  KtOutMin=[]  KtOutMax=[]  IntegratorOutMin=[]  IntegratorOutMax=[]  FilterOutMin=[]  FilterOutMax=[]  SumI1OutMin=[]  SumI1OutMax=[]  SumI2OutMin=[]  SumI2OutMax=[]  SumI3OutMin=[]  SumI3OutMax=[]  SumI4OutMin=[]  SumI4OutMax=[]  SumDOutMin=[]  SumDOutMax=[]  DifferentiatorOutMin=[]  DifferentiatorOutMax=[]  FilterDiffOutCoefMin=[]  FilterDiffOutCoefMax=[]  ReciprocalOutMin=[]  ReciprocalOutMax=[]  SumDenOutMin=[]  SumDenOutMax=[]  SumNumOutMin=[]  SumNumOutMax=[]  DivideOutMin=[]  DivideOutMax=[]  UdiffTsProdOutMin=[]  UdiffTsProdOutMax=[]  NTsProdOutMin=[]  NTsProdOutMax=[]  UintegralTsProdOutMin=[]  UintegralTsProdOutMax=[]  UngainTsProdOutMin=[]  UngainTsProdOutMax=[]  ClampingZeroOutDataTypeStr=Inherit: Inherit via back propagation  ClampingZeroOutMin=[]  ClampingZeroOutMax=[]  FilterDenConstantOutDataTypeStr=Inherit: Inherit via back propagation  FilterDenConstantOutMin=[]  FilterDenConstantOutMax=[]  PCopyOutDataTypeStr=Inherit: Inherit via back propagation  PCopyOutMin=[]  PCopyOutMax=[]  NCopyOutDataTypeStr=Inherit: Inherit via back propagation  NCopyOutMin=[]  NCopyOutMax=[]  IntegratorContinuousStateAttributes=''  IntegratorStateMustResolveToSignalObject=off  IntegratorRTWStateStorageClass=Auto  FilterContinuousStateAttributes=''  FilterStateMustResolveToSignalObject=off  FilterRTWStateStorageClass=Auto  ParallelPVariant=InternalParameters  IdealPVariant=Disabled  IVariant=InternalParameters  DVariant=InternalParameters  IntegratorVariant=Continuous  SatVariant=Disabled  AWVariant=Passthrough  PCopyVariant=Disabled  TRVariant=Disabled  FdbkBlocksVariant=Forward  IdealPFdbkVariant=Disabled  SatFdbkVariant=Disabled  DerivativeFilterVariant=ContFilter  NVariant=InternalParameters  NCopyVariant=Disabled  FilterICVariant=InternalICsFilter  IntegratorICVariant=InternalICs  ExternalResetVariant=Disabled  TRSumVariant=Passthrough  SumFdbkVariant=Disabled  SumVariant=Sum_PID  TsampFilterVariant=InternalTs  TsampNgainVariant=Passthrough  TsampIntegralVariant=Disabled_SignalSpec  ExternalSaturationOutDataTypeStr=Inherit: Same as second input
  Id_ref4 : Constant  Value=Id_ref
  Inverse Park-Clarke3 : Subsystem
  PMSM AC  4 : spsPermanentMagnetSynchronousMachineLib/Permanent Magnet Synchronous Machine  NbPhases=3  FluxDistribution=Sinusoidal  RotorType=Salient-pole  MechanicalLoad=Torque Tm  PresetModel=No  ShowDetailedParameters=on  MeasurementBus=off  Resistance=Rs  Inductance=8.5e-3  dqInductances=[Ld, Lq]  La=0.000395  MachineConstant=Flux linkage established by magnets (V.s)  Flux=flux  VoltageCst=45.345  TorqueCst=0.375  Flat=120  Mechanical=[J B pole 0]  PolePairs=4  InitialConditions=[0,0, 0,0]  InitialConditions5ph=[0 0 0 0 0 0]  RefAngle=90 degrees behind phase A axis (modified Park)  IterativeDiscreteModel=Trapezoidal non iterative  TsBlock=-1  TsPowergui=0
  Scope : Scope  NumInputPorts=2
  Scope24 : Scope
  Scope25 : Scope
  Scope26 : Scope
  Scope6 : Scope  NumInputPorts=2
  Speed_Fuzzy_Control3 : Subsystem
  Subsystem4 : Subsystem
  Three-Phase V-I Measurement4 : spsThreePhaseVIMeasurementLib/Three-Phase V-I Measurement  VoltageMeasurement=phase-to-phase  SetLabelV=off  LabelV=Vabc  Vpu=off  VpuLL=off  CurrentMeasurement=yes  SetLabelI=off  LabelI=Iabc  Ipu=off  Pbase=100e6  Vbase=500e3  OutputType=Complex  PhasorSimulation=off  PSBequivalent=0
  Universal Bridge4 : spsUniversalBridgeLib/Universal Bridge  Arms=3  SnubberResistance=1e5  SnubberCapacitance=inf  Device=IGBT / Diodes  Ron=1e-3  Lon=0  ForwardVoltages="[  0  0  ]"  ForwardVoltage=0  GTOparameters=[ 10e-6 , 20e-6 ]  IGBTparameters=[ 1e-6 , 2e-6 ]  Measurements=None  Measurements_2=None  converterType=Rectifier
  Speed : Outport
  Torque : Outport  Port=2
  wires:
  Three-Phase V-I Measurement4/2 -> Demux9/1, Scope25/1
  Subsystem4/1(switches) -> Universal Bridge4/1
  FLC_q/1(Output) -> Inverse Park-Clarke3/2(Id), Scope6/1
  Three-Phase V-I Measurement4/1 -> Scope26/1
  Demux8/2 -> Torque/1
  Inverse Park-Clarke3/1(abc) -> Scope24/1, Subsystem4/1(abc)
  Bus Selector4/1 -> Demux8/1
  Speed_Fuzzy_Control3/1(Speed_Control) -> FLC_q/1(+), Scope6/2
  Demux9/2 -> Clark_Park Transformation4/2(Ib)
  [theta_flc] -> Inverse Park-Clarke3/3(theta)
  Ref/1 -> Speed_Fuzzy_Control3/2(Speed_Ref)
  Clark_Park Transformation4/1(iq) -> FLC_q/2(-)
  Gain4/1 -> Clark_Park Transformation4/4(Theta), [theta_flc]
  Demux8/1 -> Speed/1, Speed_Fuzzy_Control3/1(Speed_Motor)
  Demux9/1 -> Clark_Park Transformation4/1(Ia)
  Demux9/3 -> Clark_Park Transformation4/3(Ic)
  Clark_Park Transformation4/2(id) -> FLC_d/2(-)
  Demux8/3 -> Gain4/1
  PMSM AC  4/1 -> Bus Selector4/1
  Id_ref4/1 -> Scope/1, FLC_d/1(+)
  Load/1 -> PMSM AC  4/1
  FLC_d/1(Output) -> Scope/2, Inverse Park-Clarke3/1(Iq)
  connections:
  DC Voltage4/LConn1 -- Universal Bridge4/RConn2
  Universal Bridge4/LConn2 -- Three-Phase V-I Measurement4/LConn2
  Three-Phase V-I Measurement4/RConn2 -- PMSM AC  4/LConn2
  Universal Bridge4/LConn3 -- Three-Phase V-I Measurement4/LConn3
  DC Voltage4/RConn1 -- Universal Bridge4/RConn1
  Universal Bridge4/LConn1 -- Three-Phase V-I Measurement4/LConn1
  Three-Phase V-I Measurement4/RConn3 -- PMSM AC  4/LConn3
  Three-Phase V-I Measurement4/RConn1 -- PMSM AC  4/LConn1

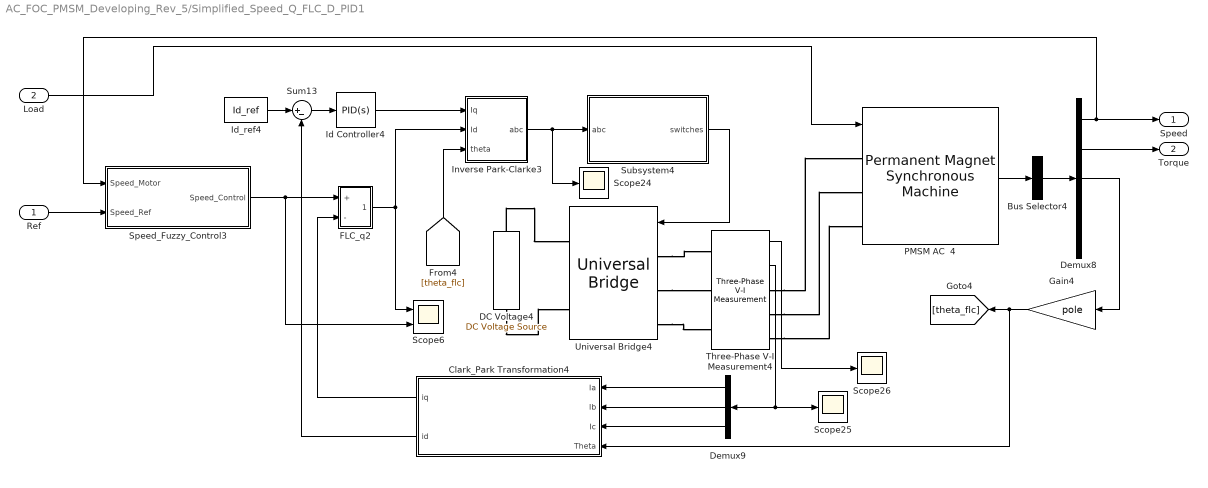
== system AC_FOC_PMSM_Developing_Rev_5/Simplified_Speed_Q_FLC_D_PID1 ==
  Ref : Inport
  Load : Inport  Port=2
  Bus Selector4 : BusSelector  OutputSignals=Rotor speed wm (rad/s),Electromagnetic torque Te (N*m),Rotor angle thetam (rad),Stator current is_q (A),Stator current is_d (A)  OutputAsBus=on
  Clark_Park Transformation4 : Subsystem
  DC Voltage4 : spsDCVoltageSourceLib/DC Voltage Source  Amplitude=600  Measurements=None
  Demux8 : Demux  Outputs=5
  Demux9 : Demux  Outputs=3
  FLC_q2 : Subsystem
  Gain4 : Gain  Gain=pole
  Id Controller4 : slpidlib/PID Controller  Controller=PID  Form=Parallel  TimeDomain=Continuous-time  UseExternalTs=off  SampleTime=-1  IntegratorMethod=Forward Euler  FilterMethod=Forward Euler  ControllerParametersSource=internal  P=Kcq  I=Kcq/0.001  UseKiTs=off  D=0  N=100  UseFilter=on  TunerSelectOption=Transfer Function Based (PID Tuner App)  InitialConditionSource=internal  InitialConditionForIntegrator=0  InitialConditionForFilter=0  DifferentiatorICPrevScaledInput=0  ExternalReset=none  TrackingMode=off  Kt=1  LimitOutput=off  SatLimitsSource=internal  UpperSaturationLimit=inf  LowerSaturationLimit=-inf  LinearizeAsGain=on  AntiWindupMode=none  Kb=1  LimitIntegrator=off  UpperIntegratorSaturationLimit=inf  LowerIntegratorSaturationLimit=-inf  POutMin=[]  POutMax=[]  IOutMin=[]  IOutMax=[]  DOutMin=[]  DOutMax=[]  NOutMin=[]  NOutMax=[]  SumOutMin=[]  SumOutMax=[]  SaturationOutMin=[]  SaturationOutMax=[]  PParamMin=[]  PParamMax=[]  IParamMin=[]  IParamMax=[]  DParamMin=[]  DParamMax=[]  NParamMin=[]  NParamMax=[]  KbParamMin=[]  KbParamMax=[]  KtParamMin=[]  KtParamMax=[]  KbOutMin=[]  KbOutMax=[]  KtOutMin=[]  KtOutMax=[]  IntegratorOutMin=[]  IntegratorOutMax=[]  FilterOutMin=[]  FilterOutMax=[]  SumI1OutMin=[]  SumI1OutMax=[]  SumI2OutMin=[]  SumI2OutMax=[]  SumI3OutMin=[]  SumI3OutMax=[]  SumI4OutMin=[]  SumI4OutMax=[]  SumDOutMin=[]  SumDOutMax=[]  DifferentiatorOutMin=[]  DifferentiatorOutMax=[]  FilterDiffOutCoefMin=[]  FilterDiffOutCoefMax=[]  ReciprocalOutMin=[]  ReciprocalOutMax=[]  SumDenOutMin=[]  SumDenOutMax=[]  SumNumOutMin=[]  SumNumOutMax=[]  DivideOutMin=[]  DivideOutMax=[]  UdiffTsProdOutMin=[]  UdiffTsProdOutMax=[]  NTsProdOutMin=[]  NTsProdOutMax=[]  UintegralTsProdOutMin=[]  UintegralTsProdOutMax=[]  UngainTsProdOutMin=[]  UngainTsProdOutMax=[]  ClampingZeroOutDataTypeStr=Inherit: Inherit via back propagation  ClampingZeroOutMin=[]  ClampingZeroOutMax=[]  FilterDenConstantOutDataTypeStr=Inherit: Inherit via back propagation  FilterDenConstantOutMin=[]  FilterDenConstantOutMax=[]  PCopyOutDataTypeStr=Inherit: Inherit via back propagation  PCopyOutMin=[]  PCopyOutMax=[]  NCopyOutDataTypeStr=Inherit: Inherit via back propagation  NCopyOutMin=[]  NCopyOutMax=[]  IntegratorContinuousStateAttributes=''  IntegratorStateMustResolveToSignalObject=off  IntegratorRTWStateStorageClass=Auto  FilterContinuousStateAttributes=''  FilterStateMustResolveToSignalObject=off  FilterRTWStateStorageClass=Auto  ParallelPVariant=InternalParameters  IdealPVariant=Disabled  IVariant=InternalParameters  DVariant=InternalParameters  IntegratorVariant=Continuous  SatVariant=Disabled  AWVariant=Passthrough  PCopyVariant=Disabled  TRVariant=Disabled  FdbkBlocksVariant=Forward  IdealPFdbkVariant=Disabled  SatFdbkVariant=Disabled  DerivativeFilterVariant=ContFilter  NVariant=InternalParameters  NCopyVariant=Disabled  FilterICVariant=InternalICsFilter  IntegratorICVariant=InternalICs  ExternalResetVariant=Disabled  TRSumVariant=Passthrough  SumFdbkVariant=Disabled  SumVariant=Sum_PID  TsampFilterVariant=InternalTs  TsampNgainVariant=Passthrough  TsampIntegralVariant=Disabled_SignalSpec  ExternalSaturationOutDataTypeStr=Inherit: Same as second input
  Id_ref4 : Constant  Value=Id_ref
  Inverse Park-Clarke3 : Subsystem
  PMSM AC  4 : spsPermanentMagnetSynchronousMachineLib/Permanent Magnet Synchronous Machine  NbPhases=3  FluxDistribution=Sinusoidal  RotorType=Salient-pole  MechanicalLoad=Torque Tm  PresetModel=No  ShowDetailedParameters=on  MeasurementBus=off  Resistance=Rs  Inductance=8.5e-3  dqInductances=[Ld, Lq]  La=0.000395  MachineConstant=Flux linkage established by magnets (V.s)  Flux=flux  VoltageCst=45.345  TorqueCst=0.375  Flat=120  Mechanical=[J B pole 0]  PolePairs=4  InitialConditions=[0,0, 0,0]  InitialConditions5ph=[0 0 0 0 0 0]  RefAngle=90 degrees behind phase A axis (modified Park)  IterativeDiscreteModel=Trapezoidal non iterative  TsBlock=-1  TsPowergui=0
  Scope24 : Scope
  Scope25 : Scope
  Scope26 : Scope
  Scope6 : Scope  NumInputPorts=2
  Speed_Fuzzy_Control3 : Subsystem
  Subsystem4 : Subsystem
  Sum13 : Sum  Inputs=|+-
  Three-Phase V-I Measurement4 : spsThreePhaseVIMeasurementLib/Three-Phase V-I Measurement  VoltageMeasurement=phase-to-phase  SetLabelV=off  LabelV=Vabc  Vpu=off  VpuLL=off  CurrentMeasurement=yes  SetLabelI=off  LabelI=Iabc  Ipu=off  Pbase=100e6  Vbase=500e3  OutputType=Complex  PhasorSimulation=off  PSBequivalent=0
  Universal Bridge4 : spsUniversalBridgeLib/Universal Bridge  Arms=3  SnubberResistance=1e5  SnubberCapacitance=inf  Device=IGBT / Diodes  Ron=1e-3  Lon=0  ForwardVoltages="[  0  0  ]"  ForwardVoltage=0  GTOparameters=[ 10e-6 , 20e-6 ]  IGBTparameters=[ 1e-6 , 2e-6 ]  Measurements=None  Measurements_2=None  converterType=Rectifier
  Speed : Outport
  Torque : Outport  Port=2
  wires:
  Three-Phase V-I Measurement4/2 -> Demux9/1, Scope25/1
  Id Controller4/1 -> Inverse Park-Clarke3/1(Iq)
  Subsystem4/1(switches) -> Universal Bridge4/1
  Sum13/1 -> Id Controller4/1
  FLC_q2/1(Output) -> Inverse Park-Clarke3/2(Id), Scope6/1
  Three-Phase V-I Measurement4/1 -> Scope26/1
  Demux8/2 -> Torque/1
  Inverse Park-Clarke3/1(abc) -> Scope24/1, Subsystem4/1(abc)
  Bus Selector4/1 -> Demux8/1
  Speed_Fuzzy_Control3/1(Speed_Control) -> FLC_q2/1(+), Scope6/2
  Demux9/2 -> Clark_Park Transformation4/2(Ib)
  [theta_flc] -> Inverse Park-Clarke3/3(theta)
  Ref/1 -> Speed_Fuzzy_Control3/2(Speed_Ref)
  Clark_Park Transformation4/1(iq) -> FLC_q2/2(-)
  Gain4/1 -> Clark_Park Transformation4/4(Theta), [theta_flc]
  Demux8/1 -> Speed/1, Speed_Fuzzy_Control3/1(Speed_Motor)
  Demux9/1 -> Clark_Park Transformation4/1(Ia)
  Demux9/3 -> Clark_Park Transformation4/3(Ic)
  Clark_Park Transformation4/2(id) -> Sum13/2
  Demux8/3 -> Gain4/1
  PMSM AC  4/1 -> Bus Selector4/1
  Id_ref4/1 -> Sum13/1
  Load/1 -> PMSM AC  4/1
  connections:
  DC Voltage4/LConn1 -- Universal Bridge4/RConn2
  Universal Bridge4/LConn2 -- Three-Phase V-I Measurement4/LConn2
  Three-Phase V-I Measurement4/RConn2 -- PMSM AC  4/LConn2
  Universal Bridge4/LConn3 -- Three-Phase V-I Measurement4/LConn3
  DC Voltage4/RConn1 -- Universal Bridge4/RConn1
  Universal Bridge4/LConn1 -- Three-Phase V-I Measurement4/LConn1
  Three-Phase V-I Measurement4/RConn3 -- PMSM AC  4/LConn3
  Three-Phase V-I Measurement4/RConn1 -- PMSM AC  4/LConn1

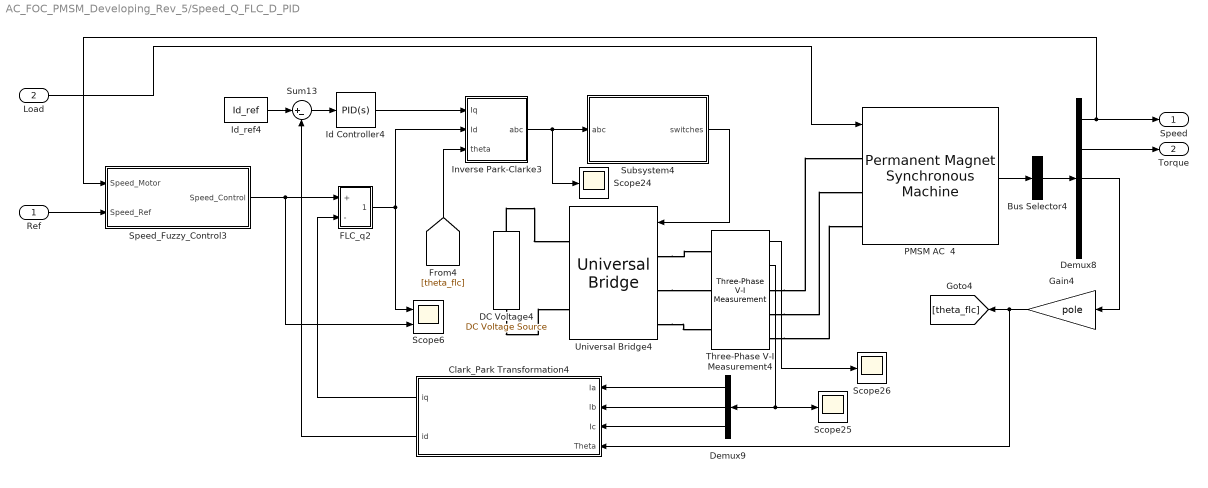
== system AC_FOC_PMSM_Developing_Rev_5/Speed_Q_FLC_D_PID ==
  Ref : Inport
  Load : Inport  Port=2
  Bus Selector4 : BusSelector  OutputSignals=Rotor speed wm (rad/s),Electromagnetic torque Te (N*m),Rotor angle thetam (rad),Stator current is_q (A),Stator current is_d (A)  OutputAsBus=on
  Clark_Park Transformation4 : Subsystem
  DC Voltage4 : spsDCVoltageSourceLib/DC Voltage Source  Amplitude=600  Measurements=None
  Demux8 : Demux  Outputs=5
  Demux9 : Demux  Outputs=3
  FLC_q2 : Subsystem
  Gain4 : Gain  Gain=pole
  Id Controller4 : slpidlib/PID Controller  Controller=PID  Form=Parallel  TimeDomain=Continuous-time  UseExternalTs=off  SampleTime=-1  IntegratorMethod=Forward Euler  FilterMethod=Forward Euler  ControllerParametersSource=internal  P=Kcq  I=Kcq/0.001  UseKiTs=off  D=0  N=100  UseFilter=on  TunerSelectOption=Transfer Function Based (PID Tuner App)  InitialConditionSource=internal  InitialConditionForIntegrator=0  InitialConditionForFilter=0  DifferentiatorICPrevScaledInput=0  ExternalReset=none  TrackingMode=off  Kt=1  LimitOutput=off  SatLimitsSource=internal  UpperSaturationLimit=inf  LowerSaturationLimit=-inf  LinearizeAsGain=on  AntiWindupMode=none  Kb=1  LimitIntegrator=off  UpperIntegratorSaturationLimit=inf  LowerIntegratorSaturationLimit=-inf  POutMin=[]  POutMax=[]  IOutMin=[]  IOutMax=[]  DOutMin=[]  DOutMax=[]  NOutMin=[]  NOutMax=[]  SumOutMin=[]  SumOutMax=[]  SaturationOutMin=[]  SaturationOutMax=[]  PParamMin=[]  PParamMax=[]  IParamMin=[]  IParamMax=[]  DParamMin=[]  DParamMax=[]  NParamMin=[]  NParamMax=[]  KbParamMin=[]  KbParamMax=[]  KtParamMin=[]  KtParamMax=[]  KbOutMin=[]  KbOutMax=[]  KtOutMin=[]  KtOutMax=[]  IntegratorOutMin=[]  IntegratorOutMax=[]  FilterOutMin=[]  FilterOutMax=[]  SumI1OutMin=[]  SumI1OutMax=[]  SumI2OutMin=[]  SumI2OutMax=[]  SumI3OutMin=[]  SumI3OutMax=[]  SumI4OutMin=[]  SumI4OutMax=[]  SumDOutMin=[]  SumDOutMax=[]  DifferentiatorOutMin=[]  DifferentiatorOutMax=[]  FilterDiffOutCoefMin=[]  FilterDiffOutCoefMax=[]  ReciprocalOutMin=[]  ReciprocalOutMax=[]  SumDenOutMin=[]  SumDenOutMax=[]  SumNumOutMin=[]  SumNumOutMax=[]  DivideOutMin=[]  DivideOutMax=[]  UdiffTsProdOutMin=[]  UdiffTsProdOutMax=[]  NTsProdOutMin=[]  NTsProdOutMax=[]  UintegralTsProdOutMin=[]  UintegralTsProdOutMax=[]  UngainTsProdOutMin=[]  UngainTsProdOutMax=[]  ClampingZeroOutDataTypeStr=Inherit: Inherit via back propagation  ClampingZeroOutMin=[]  ClampingZeroOutMax=[]  FilterDenConstantOutDataTypeStr=Inherit: Inherit via back propagation  FilterDenConstantOutMin=[]  FilterDenConstantOutMax=[]  PCopyOutDataTypeStr=Inherit: Inherit via back propagation  PCopyOutMin=[]  PCopyOutMax=[]  NCopyOutDataTypeStr=Inherit: Inherit via back propagation  NCopyOutMin=[]  NCopyOutMax=[]  IntegratorContinuousStateAttributes=''  IntegratorStateMustResolveToSignalObject=off  IntegratorRTWStateStorageClass=Auto  FilterContinuousStateAttributes=''  FilterStateMustResolveToSignalObject=off  FilterRTWStateStorageClass=Auto  ParallelPVariant=InternalParameters  IdealPVariant=Disabled  IVariant=InternalParameters  DVariant=InternalParameters  IntegratorVariant=Continuous  SatVariant=Disabled  AWVariant=Passthrough  PCopyVariant=Disabled  TRVariant=Disabled  FdbkBlocksVariant=Forward  IdealPFdbkVariant=Disabled  SatFdbkVariant=Disabled  DerivativeFilterVariant=ContFilter  NVariant=InternalParameters  NCopyVariant=Disabled  FilterICVariant=InternalICsFilter  IntegratorICVariant=InternalICs  ExternalResetVariant=Disabled  TRSumVariant=Passthrough  SumFdbkVariant=Disabled  SumVariant=Sum_PID  TsampFilterVariant=InternalTs  TsampNgainVariant=Passthrough  TsampIntegralVariant=Disabled_SignalSpec  ExternalSaturationOutDataTypeStr=Inherit: Same as second input
  Id_ref4 : Constant  Value=Id_ref
  Inverse Park-Clarke3 : Subsystem
  PMSM AC  4 : spsPermanentMagnetSynchronousMachineLib/Permanent Magnet Synchronous Machine  NbPhases=3  FluxDistribution=Sinusoidal  RotorType=Salient-pole  MechanicalLoad=Torque Tm  PresetModel=No  ShowDetailedParameters=on  MeasurementBus=off  Resistance=Rs  Inductance=8.5e-3  dqInductances=[Ld, Lq]  La=0.000395  MachineConstant=Flux linkage established by magnets (V.s)  Flux=flux  VoltageCst=45.345  TorqueCst=0.375  Flat=120  Mechanical=[J B pole 0]  PolePairs=4  InitialConditions=[0,0, 0,0]  InitialConditions5ph=[0 0 0 0 0 0]  RefAngle=90 degrees behind phase A axis (modified Park)  IterativeDiscreteModel=Trapezoidal non iterative  TsBlock=-1  TsPowergui=0
  Scope24 : Scope
  Scope25 : Scope
  Scope26 : Scope
  Scope6 : Scope  NumInputPorts=2
  Speed_Fuzzy_Control3 : Subsystem
  Subsystem4 : Subsystem
  Sum13 : Sum  Inputs=|+-
  Three-Phase V-I Measurement4 : spsThreePhaseVIMeasurementLib/Three-Phase V-I Measurement  VoltageMeasurement=phase-to-phase  SetLabelV=off  LabelV=Vabc  Vpu=off  VpuLL=off  CurrentMeasurement=yes  SetLabelI=off  LabelI=Iabc  Ipu=off  Pbase=100e6  Vbase=500e3  OutputType=Complex  PhasorSimulation=off  PSBequivalent=0
  Universal Bridge4 : spsUniversalBridgeLib/Universal Bridge  Arms=3  SnubberResistance=1e5  SnubberCapacitance=inf  Device=IGBT / Diodes  Ron=1e-3  Lon=0  ForwardVoltages="[  0  0  ]"  ForwardVoltage=0  GTOparameters=[ 10e-6 , 20e-6 ]  IGBTparameters=[ 1e-6 , 2e-6 ]  Measurements=None  Measurements_2=None  converterType=Rectifier
  Speed : Outport
  Torque : Outport  Port=2
  wires:
  Three-Phase V-I Measurement4/2 -> Demux9/1, Scope25/1
  Id Controller4/1 -> Inverse Park-Clarke3/1(Iq)
  Subsystem4/1(switches) -> Universal Bridge4/1
  Sum13/1 -> Id Controller4/1
  FLC_q2/1(Output) -> Inverse Park-Clarke3/2(Id), Scope6/1
  Three-Phase V-I Measurement4/1 -> Scope26/1
  Demux8/2 -> Torque/1
  Inverse Park-Clarke3/1(abc) -> Scope24/1, Subsystem4/1(abc)
  Bus Selector4/1 -> Demux8/1
  Speed_Fuzzy_Control3/1(Speed_Control) -> FLC_q2/1(+), Scope6/2
  Demux9/2 -> Clark_Park Transformation4/2(Ib)
  [theta_flc] -> Inverse Park-Clarke3/3(theta)
  Ref/1 -> Speed_Fuzzy_Control3/2(Speed_Ref)
  Clark_Park Transformation4/1(iq) -> FLC_q2/2(-)
  Gain4/1 -> Clark_Park Transformation4/4(Theta), [theta_flc]
  Demux8/1 -> Speed/1, Speed_Fuzzy_Control3/1(Speed_Motor)
  Demux9/1 -> Clark_Park Transformation4/1(Ia)
  Demux9/3 -> Clark_Park Transformation4/3(Ic)
  Clark_Park Transformation4/2(id) -> Sum13/2
  Demux8/3 -> Gain4/1
  PMSM AC  4/1 -> Bus Selector4/1
  Id_ref4/1 -> Sum13/1
  Load/1 -> PMSM AC  4/1
  connections:
  DC Voltage4/LConn1 -- Universal Bridge4/RConn2
  Universal Bridge4/LConn2 -- Three-Phase V-I Measurement4/LConn2
  Three-Phase V-I Measurement4/RConn2 -- PMSM AC  4/LConn2
  Universal Bridge4/LConn3 -- Three-Phase V-I Measurement4/LConn3
  DC Voltage4/RConn1 -- Universal Bridge4/RConn1
  Universal Bridge4/LConn1 -- Three-Phase V-I Measurement4/LConn1
  Three-Phase V-I Measurement4/RConn3 -- PMSM AC  4/LConn3
  Three-Phase V-I Measurement4/RConn1 -- PMSM AC  4/LConn1

== system AC_FOC_PMSM_Developing_Rev_5/FLC/Clark_Park Transformation4 ==
  Ia : Inport
  Ib : Inport  Port=2
  Ic : Inport  Port=3
  Theta : Inport  Port=4
  Gain : Gain  Gain=2/3
  Gain2 : Gain  Gain=-2/3
  Mux : Mux
  "iabc -> id" : Fcn  Expr=u(1) * sin(u(4)) + u(2) *sin(u(4) - 2*pi/3) + u(3)*sin(u(4)+2*pi/3)
  "iabc -> iq" : Fcn  Expr=u(1) * cos(u(4)) + u(2) *cos(u(4) - 2*pi/3) + u(3)*cos(u(4)+2*pi/3)
  iq : Outport
  id : Outport  Port=2
  wires:
  Gain2/1 -> id/1  "id"
  Gain/1 -> iq/1  "iq"
  "iabc -> id"/1 -> Gain2/1
  "iabc -> iq"/1 -> Gain/1
  Mux/1 -> "iabc -> iq"/1, "iabc -> id"/1
  Ia/1 -> Mux/1
  Ib/1 -> Mux/2
  Ic/1 -> Mux/3
  Theta/1 -> Mux/4

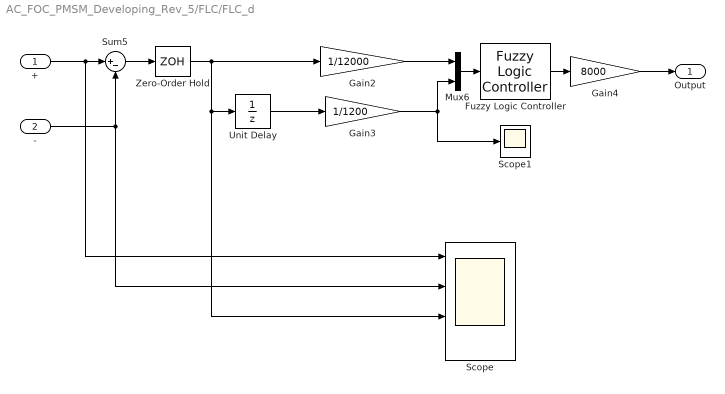
== system AC_FOC_PMSM_Developing_Rev_5/FLC/FLC_d ==
  + : Inport
  - : Inport  Port=2
  Fuzzy Logic Controller : fuzblock/Fuzzy Logic  Controller  FIS='FOC_PMSM_25.fis'  OutputSampleNumber=101  DataType=double  FuzzifiedInputs=off  RuleFiringStrengths=off  RuleOutputs=off  AggregatedOutputs=off  SimulateUsing=Interpreted execution  OutOfRangeInputValueMessage=warning  NoRuleFiredMessage=warning  EmptyOutputFuzzySetMessage=warning
  Gain2 : Gain  Gain=1/12000
  Gain3 : Gain  Gain=1/1200
  Gain4 : Gain  Gain=8000
  Mux6 : Mux  Inputs=2
  Scope : Scope  NumInputPorts=4
  Scope1 : Scope
  Sum5 : Sum  Inputs=|+-
  Unit Delay : UnitDelay  SampleTime=-1  HasFrameUpgradeWarning=on
  Zero-Order Hold : ZeroOrderHold  SampleTime=-1
  Output : Outport
  wires:
  Fuzzy Logic Controller/1 -> Gain4/1
  Mux6/1 -> Fuzzy Logic Controller/1
  Gain2/1 -> Mux6/1
  Gain3/1 -> Scope1/1, Mux6/2
  Gain4/1 -> Output/1
  Sum5/1 -> Zero-Order Hold/1
  -/1 -> Scope/2, Sum5/2
  +/1 -> Scope/1, Sum5/1
  Zero-Order Hold/1 -> Gain2/1, Scope/3, Unit Delay/1
  Unit Delay/1 -> Gain3/1
